simulink model "Esimerkki"  (R2017b)
settings: Solver=VariableStepAuto  StartTime=0.0  StopTime=100.0  RelTol=1e-3
libraries: simulink x1
settings Model: Creator=Timo Järvinen  LastModifiedBy=Timo Järvinen

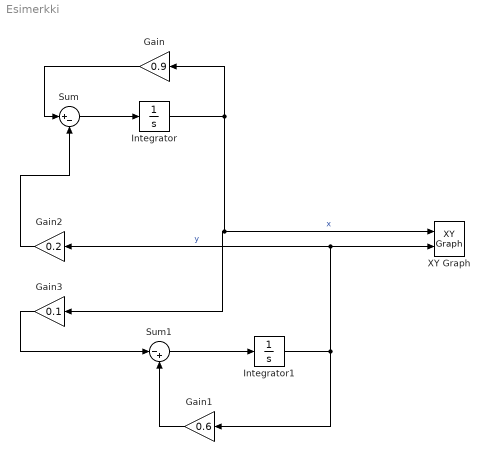
== system Esimerkki ==
  Gain : Gain  Gain=0.9
  Gain1 : Gain  Gain=0.6
  Gain2 : Gain  Gain=0.2
  Gain3 : Gain  Gain=0.1
  Integrator : Integrator  InitialCondition=1
  Integrator1 : Integrator  InitialCondition=2
  Sum : Sum  Inputs=|+-
  Sum1 : Sum  Inputs=|-+
  XY Graph : simulink/Sinks/XY Graph  xmin=0  xmax=150  ymin=0  ymax=150  st=-1
  wires:
  Integrator/1 -> Gain/1, Gain3/1, XY Graph/1  "x"
  Sum/1 -> Integrator/1
  Gain/1 -> Sum/1
  Integrator1/1 -> Gain2/1, XY Graph/2, Gain1/1  "y"
  Gain2/1 -> Sum/2
  Sum1/1 -> Integrator1/1
  Gain1/1 -> Sum1/2
  Gain3/1 -> Sum1/1
